simulink subsystem "sensors"  (R2021b)
settings: Solver=VariableStepAuto  StartTime=0.0  StopTime=10.0  RelTol=1e-3
libraries: simulink x1
settings Model: Creator=ze  LastModifiedBy=ze

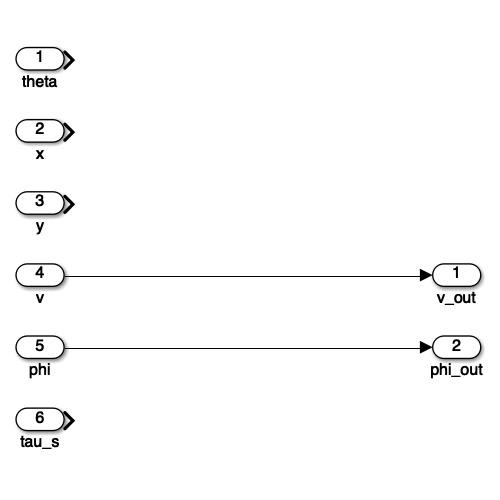
[thumbnail: Simulink's stored preview of the top-level diagram]
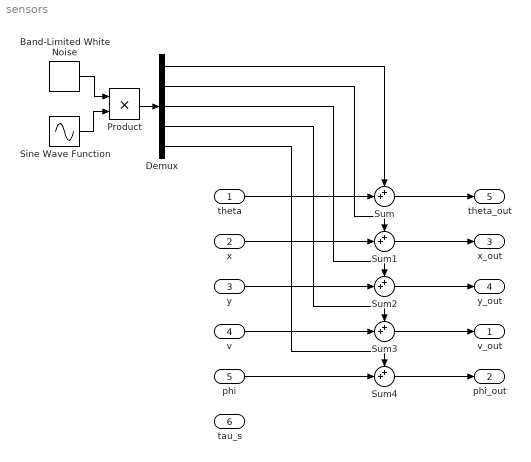
== system sensors ==
  theta : Inport
  x : Inport  Port=2
  y : Inport  Port=3
  v : Inport  Port=4
  phi : Inport  Port=5
  tau_s : Inport  Port=6
  Band-Limited White Noise : simulink/Sources/Band-Limited White Noise  Cov=[0, 0, 0, 0, 0]  Ts=0.1  seed=[23341]
  Demux : Demux  Outputs=5
  Product : Product
  Sine Wave Function : Sin  Frequency=0  SampleTime=0
  Sum{,1..4} (5 alike) : Sum  Inputs=++|
  v_out : Outport
  phi_out : Outport  Port=2
  x_out : Outport  Port=3
  y_out : Outport  Port=4
  theta_out : Outport  Port=5
  wires:
  Band-Limited White Noise/1 -> Product/1
  Sine Wave Function/1 -> Product/2
  Product/1 -> Demux/1
  Sum/1 -> theta_out/1
  Sum1/1 -> x_out/1
  Sum2/1 -> y_out/1
  Sum3/1 -> v_out/1
  Sum4/1 -> phi_out/1
  Demux/1 -> Sum/1
  Demux/2 -> Sum1/1
  Demux/3 -> Sum2/1
  Demux/4 -> Sum3/1
  Demux/5 -> Sum4/1
  theta/1 -> Sum/2
  x/1 -> Sum1/2
  y/1 -> Sum2/2
  v/1 -> Sum3/2
  phi/1 -> Sum4/2
